simulink model "model"  (R2018b)
settings: Solver=VariableStepAuto  StartTime=0.0  StopTime=10.0  RelTol=1e-3
settings Model: Creator=computer  LastModifiedBy=computer

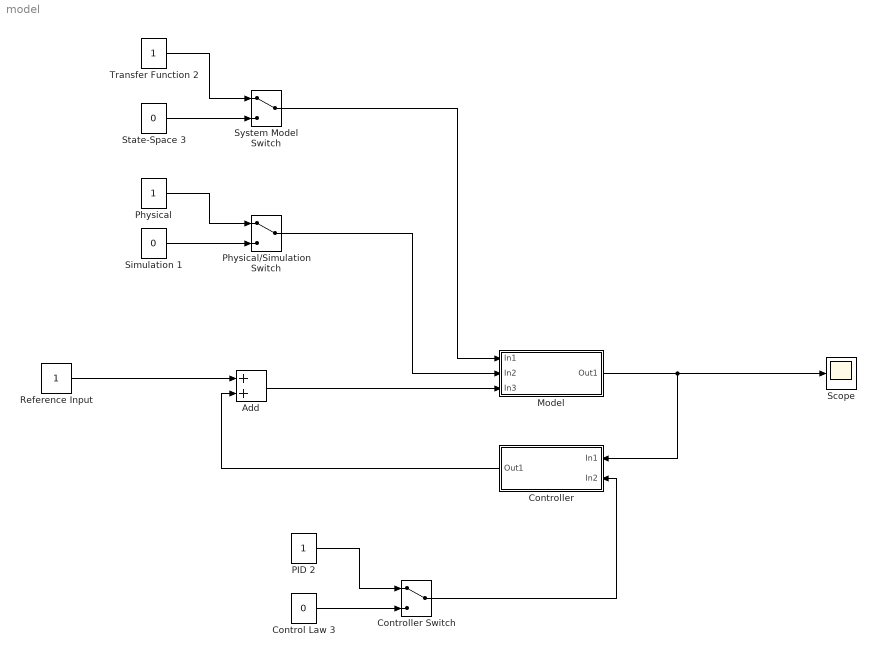
== system model ==
  Add : Sum
  Control Law 3 : Constant  Value=0
  Controller : Subsystem
  Controller Switch : ManualSwitch
  Model : Subsystem
  PID 2 : Constant
  "Physical " : Constant
  Physical/Simulation Switch : ManualSwitch
  Reference Input : Constant
  Scope : Scope
  Simulation 1 : Constant  Value=0
  State-Space 3 : Constant  Value=0
  System Model Switch : ManualSwitch
  Transfer Function 2 : Constant
  wires:
  Simulation 1/1 -> Physical/Simulation Switch/2
  "Physical "/1 -> Physical/Simulation Switch/1
  Control Law 3/1 -> Controller Switch/2
  PID 2/1 -> Controller Switch/1
  State-Space 3/1 -> System Model Switch/2
  Transfer Function 2/1 -> System Model Switch/1
  Reference Input/1 -> Add/1
  Add/1 -> Model/3(In3)
  Physical/Simulation Switch/1 -> Model/2(In2)
  System Model Switch/1 -> Model/1(In1)
  Model/1(Out1) -> Controller/1(In1), Scope/1
  Controller/1(Out1) -> Add/2
  Controller Switch/1 -> Controller/2(In2)

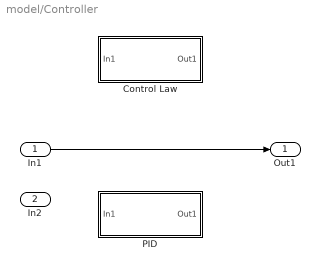
== system model/Controller ==
  In1 : Inport
  In2 : Inport  Port=2
  Control Law : Subsystem
  PID : Subsystem
  Out1 : Outport
  wires:
  In1/1 -> Out1/1

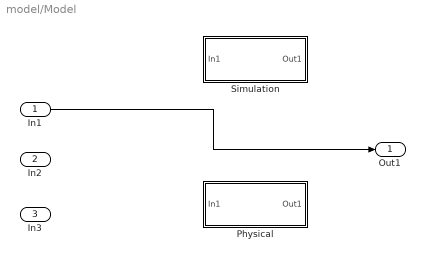
== system model/Model ==
  In1 : Inport
  In2 : Inport  Port=2
  In3 : Inport  Port=3
  Physical : Subsystem
  Simulation : Subsystem
  Out1 : Outport
  wires:
  In1/1 -> Out1/1

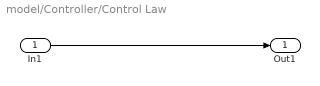
== system model/Controller/Control Law ==
  In1 : Inport
  Out1 : Outport
  wires:
  In1/1 -> Out1/1

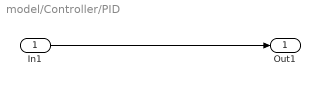
== system model/Controller/PID ==
  In1 : Inport
  Out1 : Outport
  wires:
  In1/1 -> Out1/1

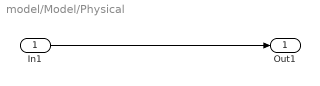
== system model/Model/Physical ==
  In1 : Inport
  Out1 : Outport
  wires:
  In1/1 -> Out1/1

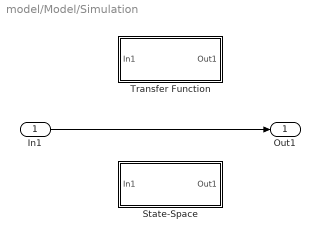
== system model/Model/Simulation ==
  In1 : Inport
  State-Space : Subsystem
  Transfer Function : Subsystem
  Out1 : Outport
  wires:
  In1/1 -> Out1/1

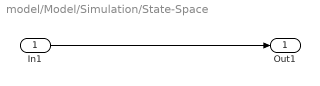
== system model/Model/Simulation/State-Space ==
  In1 : Inport
  Out1 : Outport
  wires:
  In1/1 -> Out1/1

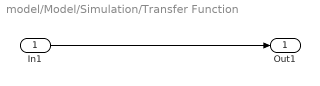
== system model/Model/Simulation/Transfer Function ==
  In1 : Inport
  Out1 : Outport
  wires:
  In1/1 -> Out1/1
